simulink model "pwm41"  (Simulink 6.3)
settings: Solver=ode45  StartTime=0  StopTime=1  MaxStep=1e-6  RelTol=1e-3
undefined symbols (not defined in the file): gcbh, powericon
libraries: powerlib x9, simulink_extras x1, simulink x1
settings Model: LastModifiedBy=zhengchunmao  StrictBusMsg=None
settings DataIOCC: LimitDataPoints=off  SignalLoggingName=sigsOut
settings DebuggingCC: SolverPrmCheckMsg=none
settings HardwareCC: TargetUnknown=on

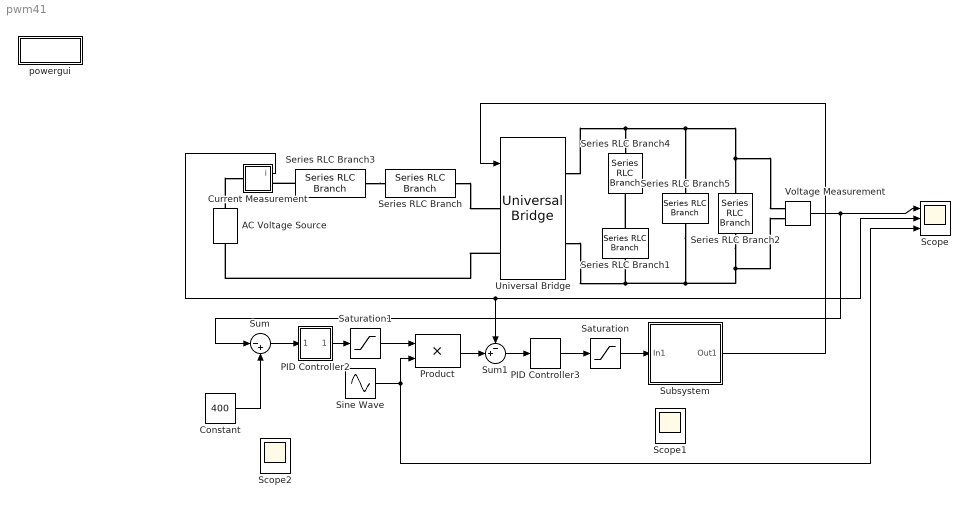
== system pwm41 ==
  AC Voltage Source : powerlib/Electrical Sources/AC Voltage Source  Description=source block  Orientation=up  Amplitude=311.08  Phase=0  Frequency=50  SampleTime=0  Measurements=None
      settings: AttributesFormatString=\n
  Constant : Constant  Value=400
  Current Measurement : Subsystem  Tag=PoWeRsYsTeMmEaSuReMeNt  AncestorBlock=powerlib/Measurements/Current Measurement  LoadFcn=powericon('psbloadfunction',gcbh,'Measurement Block','');  InitFcn=powericon('psbloadfunction',gcbh,'InitFcnOfSPSBlocks','Measurement Block');  mask(Current Measurement){PhasorSimulation=off, OutputType=Magnitude, PSBequivalent=0}
      mask prompts: PhasorSimulation "Phasor simulation"; OutputType "Output signal :"; PSBequivalent "Equivalent circuit"
      mask help: Ideal current measurement.
      mask init:
      | switch OutputType
      | case 1
      |     OutputSelection = 1;
      |     NormalMode = 2;
      |     PhasorMode = 1;
      | case 2
      |     OutputSelection =[2,3];
      |     NormalMode = 3;
      |     PhasorMode = [1,2];
      | case 3
      |     OutputSelection =[4,5];
      |     NormalMode = 3;
      |     PhasorMode = [1,2];
      | case 4
      |     OutputSelection =[4];
      |     NormalMode = 2;
      |     PhasorMode = 1;
      | end
      | %
      | if PhasorSimulation
      |     SelectionMode = PhasorMode;
      | else
      |     SelectionMode = NormalMode;
      | end
      settings: AttributesFormatString=\n  CopyFcn=powericon('psbloadfunction',gcbh,'Measurement Block','VerifyPhasor');  PreSaveFcn=powericon('psbloadfunction',gcbh,'ModelCloseFcn','');  CloseFcn=powericon('psbloadfunction',gcbh,'CloseFcn','');
      mask Help: web(psbhelp);
      mask StyleString: checkbox,popup(Complex|Real-Imag|Magnitude-Angle|Magnitude),edit
  PID Controller2 : Subsystem  AncestorBlock=simulink_extras/Additional Linear/PID Controller  mask(PID Controller){P=12, I=1e-3, D=0}
      mask prompts: P "Proportional:"; I "Integral:"; D "Derivative:"
      mask help:
      | Enter expressions for proportional, integral, and derivative terms.
      | P+I/s+Ds
      mask Help: This block implements a PID controller where parameters are entered for the Proportional, Integral and Derivative terms. Unmask this block to see how it works. The derivative term is implemented using a true derivative block.
      mask Display: disp('PID')
  PID Controller3 : simulink_extras/Additional Linear/PID Controller  P=267  I=1333  D=0
  Product : Product  SaturateOnIntegerOverflow=on
  Saturation : Saturate  UpperLimit=0.99  LowerLimit=-0.99
  Saturation1 : Saturate  UpperLimit=100  LowerLimit=-100
  Scope : Scope  NumInputPorts=3
      settings: YMin=168.5~-9~0.3  YMax=172.5~4~1
  Scope1 : Scope  NumInputPorts=2
      settings: YMin=-700~-110  YMax=1300~110  SaveName=ScopeData3
  Scope2 : Scope  NumInputPorts=2
      settings: YMin=25~125  YMax=275~375  SaveName=ScopeData4
  Series RLC Branch : powerlib/Elements/Series RLC Branch  PhysicalDomain=powersysdomain  SubClassName=unknown  LeftPortType=p1  RightPortType=p1  LConnTagsString=__new0  RConnTagsString=__new0  BranchType=L  Resistance=[]  Inductance=40e-3  SetiL0=off  InitialCurrent=0  Capacitance=[]  Setx0=off  InitialVoltage=0  Measurements=None
  Series RLC Branch1 : powerlib/Elements/Series RLC Branch  Orientation=down  PhysicalDomain=powersysdomain  SubClassName=unknown  LeftPortType=p1  RightPortType=p1  LConnTagsString=__new0  RConnTagsString=__new0  BranchType=C  Resistance=[]  Inductance=[]  SetiL0=off  InitialCurrent=0  Capacitance=1000e-6  Setx0=off  InitialVoltage=0  Measurements=None
  Series RLC Branch2 : powerlib/Elements/Series RLC Branch  Orientation=down  PhysicalDomain=powersysdomain  SubClassName=unknown  LeftPortType=p1  RightPortType=p1  LConnTagsString=__new0  RConnTagsString=__new0  BranchType=R  Resistance=100  Inductance=0.005  SetiL0=off  InitialCurrent=0  Capacitance=[]  Setx0=off  InitialVoltage=0  Measurements=None
  Series RLC Branch3 : powerlib/Elements/Series RLC Branch  PhysicalDomain=powersysdomain  SubClassName=unknown  LeftPortType=p1  RightPortType=p1  LConnTagsString=__new0  RConnTagsString=__new0  BranchType=R  Resistance=0.2  Inductance=0.005  SetiL0=off  InitialCurrent=0  Capacitance=[]  Setx0=off  InitialVoltage=0  Measurements=None
  Series RLC Branch4 : powerlib/Elements/Series RLC Branch  Orientation=down  PhysicalDomain=powersysdomain  SubClassName=unknown  LeftPortType=p1  RightPortType=p1  LConnTagsString=__new0  RConnTagsString=__new0  BranchType=L  Resistance=32.8  Inductance=2.5e-3  SetiL0=off  InitialCurrent=0  Capacitance=[]  Setx0=off  InitialVoltage=0  Measurements=None
  Series RLC Branch5 : powerlib/Elements/Series RLC Branch  Orientation=down  PhysicalDomain=powersysdomain  SubClassName=unknown  LeftPortType=p1  RightPortType=p1  LConnTagsString=__new0  RConnTagsString=__new0  BranchType=C  Resistance=[]  Inductance=[]  SetiL0=off  InitialCurrent=0  Capacitance=3000e-6  Setx0=off  InitialVoltage=0  Measurements=None
  Sine Wave : Sin  Frequency=2*pi*50  SampleTime=0
  Subsystem : Subsystem
  Sum : Sum  Inputs=|-+  SaturateOnIntegerOverflow=on
  Sum1 : Sum  Inputs=-+|  SaturateOnIntegerOverflow=on
  Universal Bridge : powerlib/Power Electronics/Universal Bridge  Arms=2  SnubberResistance=10000  SnubberCapacitance=0.001e-6  Device=IGBT / Diodes  Ron=0.01  Lon=0  ForwardVoltages=[1,0.8 ]  ForwardVoltage=0  GTOparameters=[ 10e-6 , 20e-6 ]  IGBTparameters=[ 1e-6 , 2e-6 ]  Measurements=Device currents  converterType=Rectifier
  Voltage Measurement : powerlib/Measurements/Voltage Measurement  Tag=PoWeRsYsTeMmEaSuReMeNt  PhasorSimulation=off  OutputType=Magnitude  PSBequivalent=0
  powergui : Subsystem  AncestorBlock=powerlib/powergui  mask(PSB option menu block){SimulationMode=Continuous, SampleTime=0, echomessages=off, x0status=blocks, Frange=[0:2:500], Ylog=off, Xlog=on, ShowGrid=off, save=off, variable=ZData, structure=, ZoomFFT=on, StartTime=0.0, cycles=1, DisplayStyle=1, fundamental=60, FreqAxis=off, MaxFrequency=1000, frequencyindice=1, frequencyindicesteady=1, RmsSteady=1, display=off, Ts=0, frequency=60, methode=off}
      mask prompts: SimulationMode "General parameter: Simulation Mode"; SampleTime "General parameter: Sample Time"; echomessages "General parameter: Echo  Messages"; x0status "Initial electrical states status"; Frange "Impedance tool: Frequency Range"; Ylog "Impedance tool: Log impedance"; Xlog "Impedance tool: log Frequency"; ShowGrid "Impedance tool: grid"; save "Impedance tool: Save Data To Workspace"; variable "Impedance tool: Variable Name"; structure "Structure Name (PSBFFTSCOPE)"; ZoomFFT "ZoomFFT (PSBFFTSCOPE)"; StartTime "Start Time (PSBFFTSCOPE)"; cycles "Cycles (PSBFFTSCOPE)"; DisplayStyle "Display style (PSBFFTSCOPE)"; fundamental "Fundamental (PSBFFTSCOPE)"; FreqAxis "Frequency Axis (PSBFFTSCOPE)"; MaxFrequency "Max Frequency (PSBFFTSCOPE)"; frequencyindice "Frequency indice  (PSBLOADFLOW)"; frequencyindicesteady "Frequency indice (STEADYSTATE)"; RmsSteady "RMS display (STEADYSTATE)"; display "Display Results"; Ts "Sample time (s):"; frequency "General parameter: phasor frequency"; methode "Phasor simulation"
      mask init:
      | powerlibroot = which('powersysdomain');
      | PSBroot = powerlibroot(1:end-16);
      | %
      | switch SimulationMode
      | 	case 1
      | 		message=sprintf('Continuous');
      | 	case 2
      |         message=sprintf('Discrete,\nTs = %.4g s.',SampleTime);
      | 	case 3
      | 		message=sprintf('Phasors');
      | end
      | if strcmp(bdroot,'powerlib')
      |   message='powergui';
      | end
      | power_initmask();
      settings: CopyFcn=powergui('Copy_Callback',gcb,0,[]);  DeleteFcn=powergui('Copy_Callback',gcb,1,[]);powergui('Close_Callback',gcb,[],[]);  ModelCloseFcn=powergui('Close_Callback',gcb,[],[]);  NameChangeFcn=handles = get_param(gcb,'UserData');if ~isempty(handles);delete(handles.powergui);end
      settings: PreSaveFcn=|
      | try
      | close(get_param(gcbh,'userdata'))
      | end
      settings: OpenFcn=|
      | if (power_openblockproxy ('secondary'))
      | powergui(gcb,'PM')
      | end;
      mask Help: web(psbhelp)
      mask StyleString: popup(Continuous|Discrete|Phasor),edit,checkbox,popup(blocks|steady|zero),edit,checkbox,checkbox,checkbox,checkbox,edit,edit,checkbox,edit,edit,edit,edit,checkbox,edit,edit,edit,edit,checkbox,edit,edit,checkbox
      mask Display: disp(message)
  wires:
  Constant/1 -> Sum/2
  Sum1/1 -> PID Controller3/1
  Sine Wave/1 -> Product/2, Scope/3
  Product/1 -> Sum1/2
  Subsystem/1(Out1) -> Universal Bridge/1
  Current Measurement/1(i) -> Sum1/1, Scope/2
  Sum/1 -> PID Controller2/1(In_1)
  PID Controller3/1 -> Saturation/1
  Saturation/1 -> Subsystem/1(In1)
  PID Controller2/1(Out_1) -> Saturation1/1
  Saturation1/1 -> Product/1
  Voltage Measurement/1 -> Scope/1, Sum/1
  connections:
  AC Voltage Source/RConn1 -- Current Measurement/LConn1
  Series RLC Branch/RConn1 -- Universal Bridge/LConn1
  Universal Bridge/LConn2 -- AC Voltage Source/LConn1
  Series RLC Branch3/LConn1 -- Current Measurement/RConn1
  Series RLC Branch3/RConn1 -- Series RLC Branch/LConn1
  Universal Bridge/RConn1 -- Series RLC Branch4/LConn1 -- Series RLC Branch5/LConn1 -- Series RLC Branch2/LConn1 -- Voltage Measurement/LConn1
  Series RLC Branch1/LConn1 -- Series RLC Branch4/RConn1
  Series RLC Branch2/RConn1 -- Series RLC Branch5/RConn1 -- Universal Bridge/RConn2 -- Series RLC Branch1/RConn1 -- Voltage Measurement/LConn2

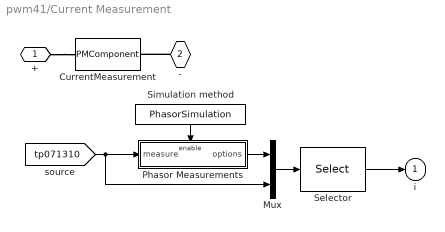
== system pwm41/Current Measurement ==
  CurrentMeasurement : PMComponent  PhysicalDomain=powersysdomain  LeftPortType=p1  RightPortType=p1  LConnTagsString=a  RConnTagsString=__new0
      mask Type: InnerPowersysBlock
  Mux : Mux  Inputs=2
  Phasor Measurements : Subsystem  TreatAsAtomicUnit=on
  Selector : Selector  Elements=SelectionMode  InputPortWidth=length(OutputSelection)+1
  Simulation method : Constant  Orientation=down  Value=PhasorSimulation
  + : PMIOPort  Port=1  Side=Left
  - : PMIOPort  Orientation=left  Port=2  Side=Right
  i : Outport  InitialOutput=0
  wires:
  Simulation method/1 -> Phasor Measurements/Enable
  Mux/1 -> Selector/1
  Phasor Measurements/1(options) -> Mux/1
  [tp071310] -> Mux/2, Phasor Measurements/1(measure)
  Selector/1 -> i/1
  connections:
  +/RConn1 -- CurrentMeasurement/LConn1
  -/RConn1 -- CurrentMeasurement/RConn1

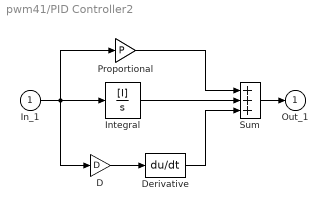
== system pwm41/PID Controller2 ==
  In_1 : Inport
  D : Gain  Gain=D  SaturateOnIntegerOverflow=on
  Derivative : Derivative
  Integral : TransferFcn  Numerator=[I]  Denominator=[1 0]
  Proportional : Gain  Gain=P  SaturateOnIntegerOverflow=on
  Sum : Sum  Inputs=+++  SaturateOnIntegerOverflow=on  InputSameDT=on
  Out_1 : Outport  InitialOutput=0
  wires:
  Proportional/1 -> Sum/1
  Integral/1 -> Sum/2
  In_1/1 -> Integral/1, Proportional/1, D/1
  Sum/1 -> Out_1/1
  D/1 -> Derivative/1
  Derivative/1 -> Sum/3

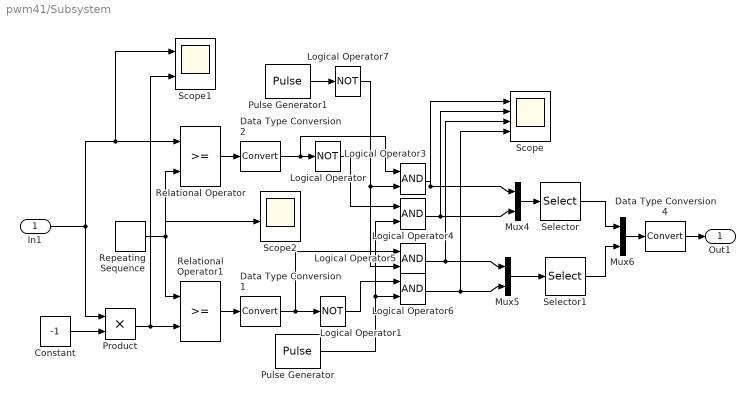
== system pwm41/Subsystem ==
  In1 : Inport
  Constant : Constant  Value=-1
  Data Type Conversion1 : DataTypeConversion  OutDataTypeMode=boolean  SaturateOnIntegerOverflow=on  RndMeth=Zero
  Data Type Conversion2 : DataTypeConversion  OutDataTypeMode=boolean  SaturateOnIntegerOverflow=on  RndMeth=Zero
  Data Type Conversion4 : DataTypeConversion  OutDataTypeMode=double  SaturateOnIntegerOverflow=on  RndMeth=Zero
  Logical Operator : Logic  Operator=NOT  AllPortsSameDT=off  OutDataTypeMode=Specify via dialog
  Logical Operator1 : Logic  Operator=NOT  AllPortsSameDT=off  OutDataTypeMode=Specify via dialog
  Logical Operator{3..6} (4 alike) : Logic  AllPortsSameDT=off  OutDataTypeMode=Specify via dialog
  Logical Operator7 : Logic  Operator=NOT  AllPortsSameDT=off  OutDataTypeMode=Specify via dialog
  Mux4 : Mux  Inputs=2
  Mux5 : Mux  Inputs=2
  Mux6 : Mux  Inputs=2
  Product : Product  RndMeth=Zero
  Pulse Generator : DiscretePulseGenerator  PulseType=Time based  Period=1/20e3  PulseWidth=50
  Pulse Generator1 : DiscretePulseGenerator  PulseType=Time based  Period=1/20e3  PulseWidth=50
  Relational Operator : RelationalOperator
  Relational Operator1 : RelationalOperator
  Repeating Sequence : simulink/Sources/Repeating Sequence  rep_seq_t=[0 0.000025 0.00005]  rep_seq_y=[0 1 0]
  Scope : Scope  NumInputPorts=4
      settings: YMin=-1~-1~-1~-1  YMax=2~2~2~2
  Scope1 : Scope  NumInputPorts=2
      settings: YMin=-1~-1  YMax=2~2  SaveName=ScopeData2
  Scope2 : Scope  NumInputPorts=4
      settings: YMin=-1~-1~-1~-1  YMax=2~2~2~2  SaveName=ScopeData5
  Selector : Selector  Elements=[1 2]  InputPortWidth=2
  Selector1 : Selector  Elements=[2 1]  InputPortWidth=2
  Out1 : Outport
  wires:
  Repeating Sequence/1 -> Relational Operator/2, Relational Operator1/1, Scope2/3
  Relational Operator/1 -> Data Type Conversion2/1
  Relational Operator1/1 -> Data Type Conversion1/1
  Product/1 -> Relational Operator1/2, Scope1/2
  In1/1 -> Product/1, Relational Operator/1, Scope1/1
  Data Type Conversion1/1 -> Logical Operator1/1, Logical Operator5/1
  Data Type Conversion2/1 -> Logical Operator/1, Logical Operator3/1
  Logical Operator/1 -> Logical Operator4/1
  Logical Operator1/1 -> Logical Operator6/1
  Mux5/1 -> Selector1/1
  Mux4/1 -> Selector/1
  Selector/1 -> Mux6/1
  Selector1/1 -> Mux6/2
  Mux6/1 -> Data Type Conversion4/1
  Data Type Conversion4/1 -> Out1/1
  Logical Operator6/1 -> Mux5/2, Scope/4
  Logical Operator5/1 -> Mux5/1, Scope/3
  Logical Operator4/1 -> Mux4/2, Scope/2
  Logical Operator3/1 -> Mux4/1, Scope/1
  Pulse Generator/1 -> Logical Operator4/2, Logical Operator6/2
  Pulse Generator1/1 -> Logical Operator7/1
  Logical Operator7/1 -> Logical Operator5/2, Logical Operator3/2
  Constant/1 -> Product/2

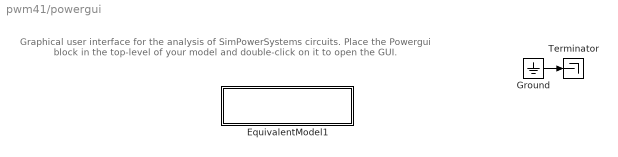
== system pwm41/powergui ==
  note: Graphical user interface for the analysis of  SimPowerSystems circuits.
      | Place the Powergui block in the top-level of your model and double-click
      | on it to open the GUI.
  EquivalentModel1 : Subsystem
      mask init:
      | SPS = get_param(gcbh,'UserData');
      | if isempty(SPS)
      |     A=0;
      |     B=0;
      |     C=0;
      |     D=0;
      |     x0=0;
      |     SwitchResistance=1;
      |     SwitchType=1;
      |     SwitchGateInitialValue=1;
      |     OutputsToResetToZero=1;
      | else
      | 	A=SPS.A;
      |     B=SPS.B;
      |     C=SPS.C;
      |     D=SPS.D;
      |     x0=SPS.x0;
      |     SwitchResistance=SPS.SwitchResistance;
      |     SwitchType=SPS.SwitchType;
      |     SwitchGateInitialValue=SPS.SwitchGateInitialValue;
      |     OutputsToResetToZero=SPS.YSwitchCurrent;
      | end
      mask Display:
      | color('blue')
      | disp('EQUIVALENT CIRCUIT')
  Ground : Ground
  Terminator : Terminator
  wires:
  Ground/1 -> Terminator/1

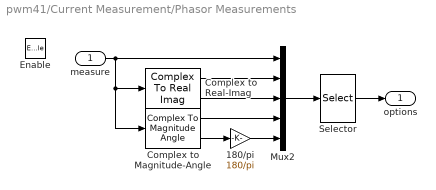
== system pwm41/Current Measurement/Phasor Measurements ==
  measure : Inport
  Enable : EnablePort
  180/pi : Gain  Gain=180/pi  SaturateOnIntegerOverflow=on
  Complex to Magnitude-Angle : ComplexToMagnitudeAngle
  Complex to Real-Imag : ComplexToRealImag
  Mux2 : Mux  Inputs=5
  Selector : Selector  Elements=OutputSelection  InputPortWidth=5
  options : Outport  InitialOutput=0
  wires:
  Mux2/1 -> Selector/1
  measure/1 -> Complex to Magnitude-Angle/1, Complex to Real-Imag/1, Mux2/1
  Complex to Real-Imag/1 -> Mux2/2
  Complex to Real-Imag/2 -> Mux2/3
  Complex to Magnitude-Angle/1 -> Mux2/4
  Complex to Magnitude-Angle/2 -> 180/pi/1
  180/pi/1 -> Mux2/5
  Selector/1 -> options/1

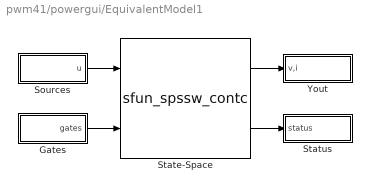
== system pwm41/powergui/EquivalentModel1 ==
  Gates : Subsystem
  Sources : Subsystem
  State-Space : S-Function  FunctionName=sfun_spssw_contc  Parameters=A, B, C, D, x0, SwitchResistance ,SwitchType, SwitchGateInitialValue, OutputsToResetToZero
  Status : Subsystem
  Yout : Subsystem
  wires:
  State-Space/1 -> Yout/1(v,i)
  State-Space/2 -> Status/1(status)
  Sources/1(u) -> State-Space/1
  Gates/1(gates) -> State-Space/2

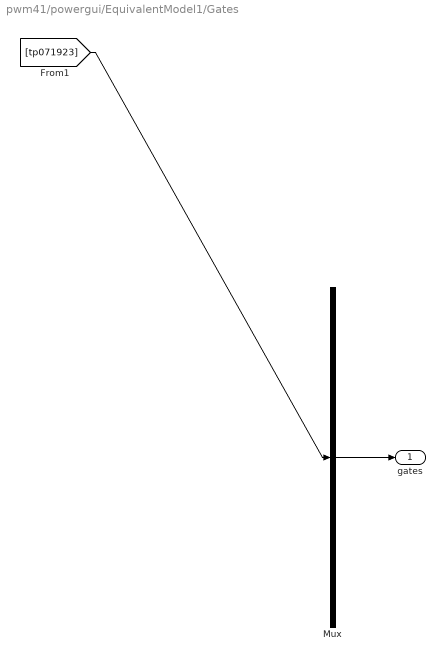
== system pwm41/powergui/EquivalentModel1/Gates ==
  Mux : Mux  Inputs=1
  gates : Outport
  wires:
  Mux/1 -> gates/1
  [tp071923] -> Mux/1

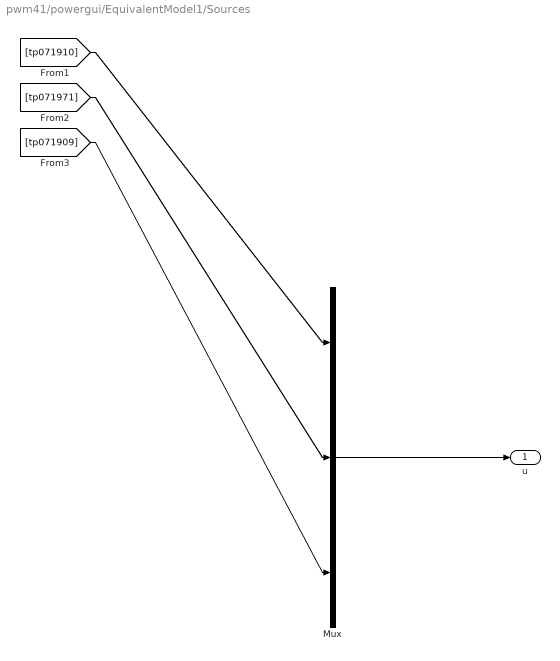
== system pwm41/powergui/EquivalentModel1/Sources ==
  Mux : Mux  Inputs=[4 1 4]
  u : Outport
  wires:
  Mux/1 -> u/1
  [tp071910] -> Mux/1
  [tp071971] -> Mux/2
  [tp071909] -> Mux/3

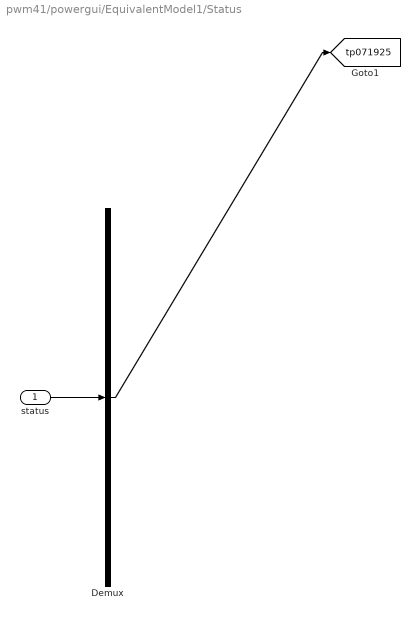
== system pwm41/powergui/EquivalentModel1/Status ==
  status : Inport
  Demux : Demux  Outputs=1
  tag scope: tp071925=global
  wires:
  status/1 -> Demux/1
  Demux/1 -> [tp071925]

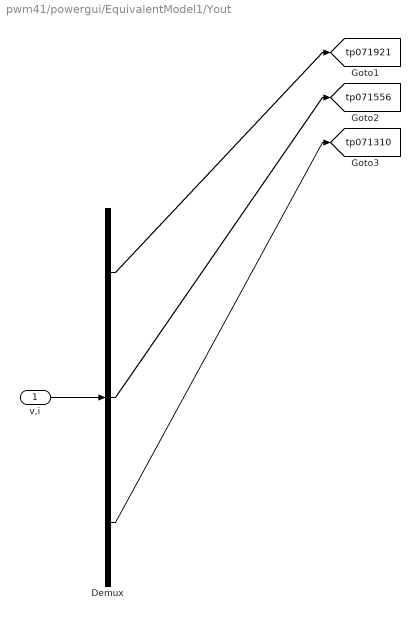
== system pwm41/powergui/EquivalentModel1/Yout ==
  v,i : Inport
  Demux : Demux  Outputs=[4 1 1]
  tag scope: tp071310=global, tp071556=global, tp071921=global
  wires:
  v,i/1 -> Demux/1
  Demux/1 -> [tp071921]
  Demux/2 -> [tp071556]
  Demux/3 -> [tp071310]
